simulink model "mat_fnetjob4"  (R2024a)
settings: Solver=VariableStepAuto  StartTime=0.0  StopTime=150  RelTol=1e-3
model workspace (MAT data in the model file):
  effi = 0.9
  g = 9.81
  m = 1300
  r_wheel = 0.3
libraries: simulink x1
settings Model: Creator=Akshata  LastModifiedBy=Akshata

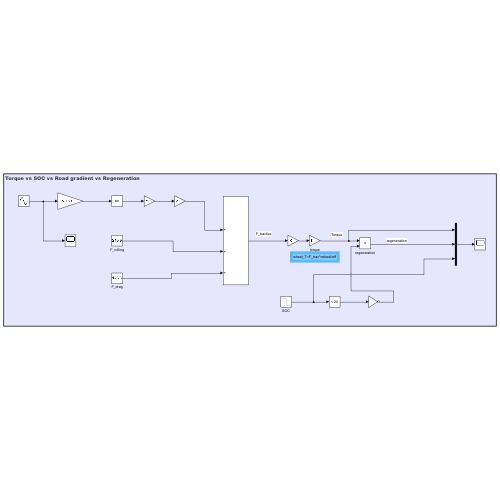
[thumbnail: Simulink's stored preview of the top-level diagram]
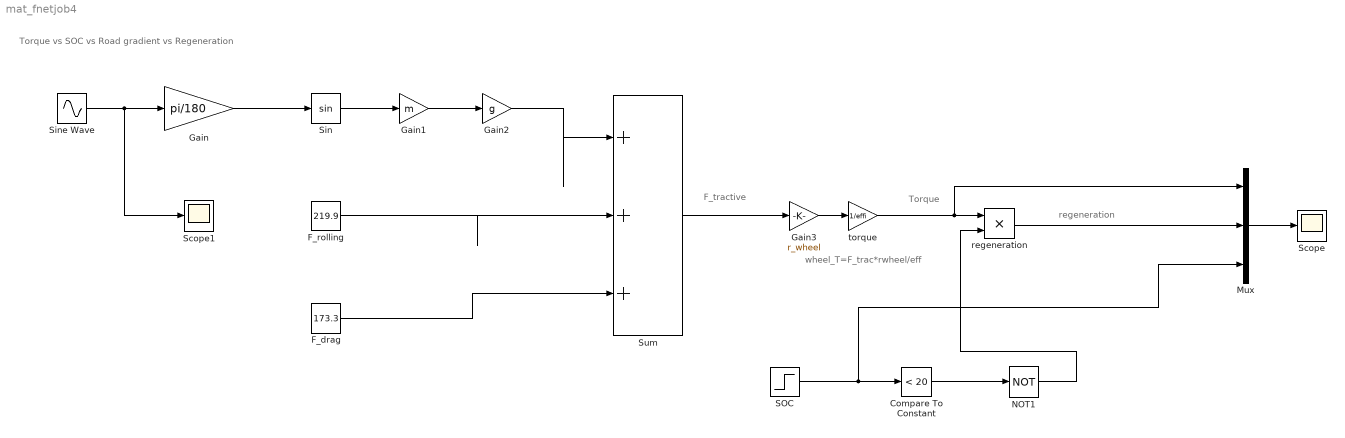
== system mat_fnetjob4 ==
  note: Torque vs SOC vs Road gradient vs Regeneration
  note: regeneration
  note: wheel_T=F_trac*rwheel/eff
  note: Torque
  note: F_tractive
  Compare To Constant : simulink/Logic and Bit Operations/Compare To Constant  relop=<  const=20  OutDataTypeStr=boolean
  F_drag : Constant  Value=173.3
  F_rolling : Constant  Value=219.9
  Gain : Gain  Gain=pi/180
  Gain1 : Gain  Gain=m
  Gain2 : Gain  Gain=g
  Gain3 : Gain  Gain=r_wheel
  Mux : Mux  Inputs=3
  NOT1 : Logic  Operator=NOT  IconShape=distinctive  AllPortsSameDT=off  OutDataTypeStr=boolean
  SOC : Step  Time=5  Before=80  After=15  SampleTime=0
  Scope : Scope
  Scope1 : Scope
  Sin : Trigonometry
  Sine Wave : Sin  Amplitude=5  Bias=5  Frequency=0.01  SampleTime=0
  Sum : Sum  Inputs=|+++
  regeneration : Product
  torque : Gain  Gain=1/effi
  wires:
  Gain/1 -> Sin/1
  Gain1/1 -> Gain2/1
  SOC/1 -> Mux/3, Compare To Constant/1
  Gain2/1 -> Sum/1
  F_rolling/1 -> Sum/2
  F_drag/1 -> Sum/3
  Sum/1 -> Gain3/1
  Gain3/1 -> torque/1
  torque/1 -> Mux/1, regeneration/1
  Compare To Constant/1 -> NOT1/1
  regeneration/1 -> Mux/2
  Sin/1 -> Gain1/1
  Sine Wave/1 -> Scope1/1, Gain/1
  NOT1/1 -> regeneration/2
  Mux/1 -> Scope/1
